simulink model "vcpinvex"  (Simulink 3.00)
settings: Solver=FixedStepDiscrete  StartTime=0.0  StopTime=499.0  RelTol=1e-3
libraries: smxl x4, simulink3 x2
settings Model: LastModifiedBy=giampiero

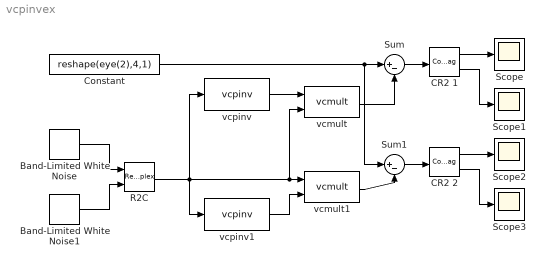
== system vcpinvex ==
  Band-Limited White Noise : simulink3/Sources/Band-Limited White Noise  Cov=[0.1]*ones(6,1)  Ts=0.1  seed=1:6
  Band-Limited White Noise1 : simulink3/Sources/Band-Limited White Noise  Cov=[0.1]*ones(6,1)  Ts=0.1  seed=7:12
  CR2 1 : ComplexToRealImag  Output=RealAndImag
  CR2 2 : ComplexToRealImag  Output=RealAndImag
  Constant : Constant  Value=reshape(eye(2),4,1)
  R2C : RealImagToComplex  Input=RealAndImag  ConstantPart=0
  Scope{,1..3} (4 alike) : Scope
      settings: TimeRange=500  YMin=-4e-015  YMax=4e-015  SaveToWorkspace=off  SaveName=ScopeData
  Sum : Sum  Inputs=|+-  SaturateOnIntegerOverflow=on
  Sum1 : Sum  Inputs=|+-  SaturateOnIntegerOverflow=on
  vcmult : smxl/Complex Matrices/vcmult  d=[2 3 2]
  vcmult1 : smxl/Complex Matrices/vcmult  d=[2 3 2]
  vcpinv : smxl/Complex Matrices/vcpinv  d=[3 2]  tol=1
  vcpinv1 : smxl/Complex Matrices/vcpinv  d=[2 3]  tol=1
  wires:
  vcpinv/1 -> vcmult/1
  Constant/1 -> Sum1/1, Sum/1
  Sum/1 -> CR2 1/1
  CR2 1/1 -> Scope/1
  CR2 1/2 -> Scope1/1
  CR2 2/1 -> Scope2/1
  CR2 2/2 -> Scope3/1
  vcmult1/1 -> Sum1/2
  Sum1/1 -> CR2 2/1
  Band-Limited White Noise/1 -> R2C/1
  Band-Limited White Noise1/1 -> R2C/2
  vcpinv1/1 -> vcmult1/2
  R2C/1 -> vcmult1/1, vcmult/2, vcpinv/1, vcpinv1/1
  vcmult/1 -> Sum/2
